simulink model "massgyro_plant"  (R2019b)
settings: Solver=VariableStepAuto  StartTime=0.0  StopTime=62  RelTol=1e-5
values from neighbouring files (symbols this model uses):
  c = 0.2    [PlantParams.mat]    (also in params.m = 0.1)
  dtheta1 = 41.8879020479    [PlantParams.mat]    (also in params.m)
  Eo = 0    [PlantParams.mat]    (also in params.m)
  g = 9.81    [PlantParams.mat]    (also in params.m)
  Id = 0.0148    [PlantParams.mat]    (also in params.m)
  J1 = 0.13138281053    [PlantParams.mat]    (also in params.m = 0.1314)
  Jz_bar = 0.0130765    [PlantParams.mat]    (also in params.m = 0.0131)
  k = 0.2    [PlantParams.mat]    (also in params.m)
  lcg = 0.269778481013    [PlantParams.mat]    (also in params.m = 0.2698)
  m = 0.158    [PlantParams.mat]    (also in params.m)
  rh = 0.37    [PlantParams.mat]    (also in params.m)
settings Model: Creator=Nilpa  LastModifiedBy=Nilpa
settings SolverCC: AlgebraicLoopSolver=LineSearch

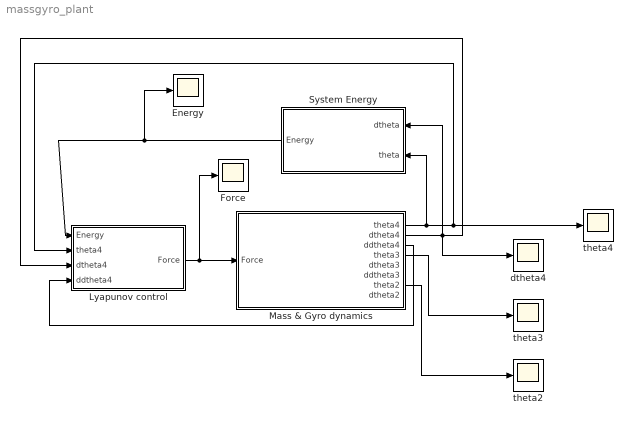
== system massgyro_plant ==
  Energy : Scope
  Force : Scope
  Lyapunov control : Subsystem
  Mass & Gyro dynamics : Subsystem
  System Energy : Subsystem
  dtheta4 : Scope
  theta2 : Scope
  theta3 : Scope
  theta4 : Scope
  wires:
  Mass & Gyro dynamics/1(theta4) -> theta4/1, Lyapunov control/2(theta4), System Energy/2(theta)
  Mass & Gyro dynamics/2(dtheta4) -> dtheta4/1, Lyapunov control/3(dtheta4), System Energy/1(dtheta)
  System Energy/1(Energy) -> Energy/1, Lyapunov control/1(Energy)
  Mass & Gyro dynamics/3(ddtheta4) -> Lyapunov control/4(ddtheta4)
  Lyapunov control/1(Force) -> Force/1, Mass & Gyro dynamics/1(Force)
  Mass & Gyro dynamics/4(theta3) -> theta3/1
  Mass & Gyro dynamics/7(theta2) -> theta2/1

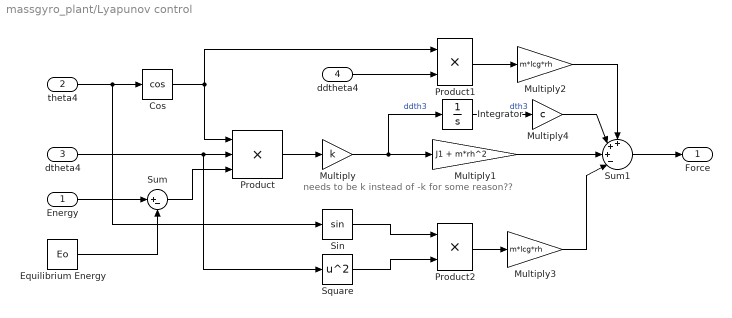
== system massgyro_plant/Lyapunov control ==
  note: needs to be k instead of -k for some reason??
  Energy : Inport
  theta4 : Inport  Port=2
  dtheta4 : Inport  Port=3
  ddtheta4 : Inport  Port=4
  Cos : Trigonometry  Operator=cos
  Equilibrium Energy : Constant  Value=Eo
  Integrator : Integrator
  Multiply : Gain  Gain=k
  Multiply1 : Gain  Gain=J1 + m*rh^2
  Multiply2 : Gain  Gain=m*lcg*rh
  Multiply3 : Gain  Gain=m*lcg*rh
  Multiply4 : Gain  Gain=c
  Product : Product  Inputs=3
  Product1 : Product
  Product2 : Product
  Sin : Trigonometry
  Square : Math  Operator=square  SignedPower=off  SaturateOnIntegerOverflow=on
  Sum : Sum  Inputs=|+-
  Sum1 : Sum  Inputs=+++-|
  Force : Outport
  wires:
  Product/1 -> Multiply/1
  theta4/1 -> Cos/1, Sin/1
  Cos/1 -> Product/1, Product1/1
  dtheta4/1 -> Product/2, Square/1
  Energy/1 -> Sum/1
  Sum/1 -> Product/3
  Equilibrium Energy/1 -> Sum/2
  Multiply/1 -> Integrator/1, Multiply1/1  "ddth3"
  Multiply1/1 -> Sum1/3
  Sum1/1 -> Force/1
  Product1/1 -> Multiply2/1
  Multiply2/1 -> Sum1/1
  Sin/1 -> Product2/1
  Square/1 -> Product2/2
  Product2/1 -> Multiply3/1
  Multiply3/1 -> Sum1/4
  ddtheta4/1 -> Product1/2
  Integrator/1 -> Multiply4/1  "dth3"
  Multiply4/1 -> Sum1/2

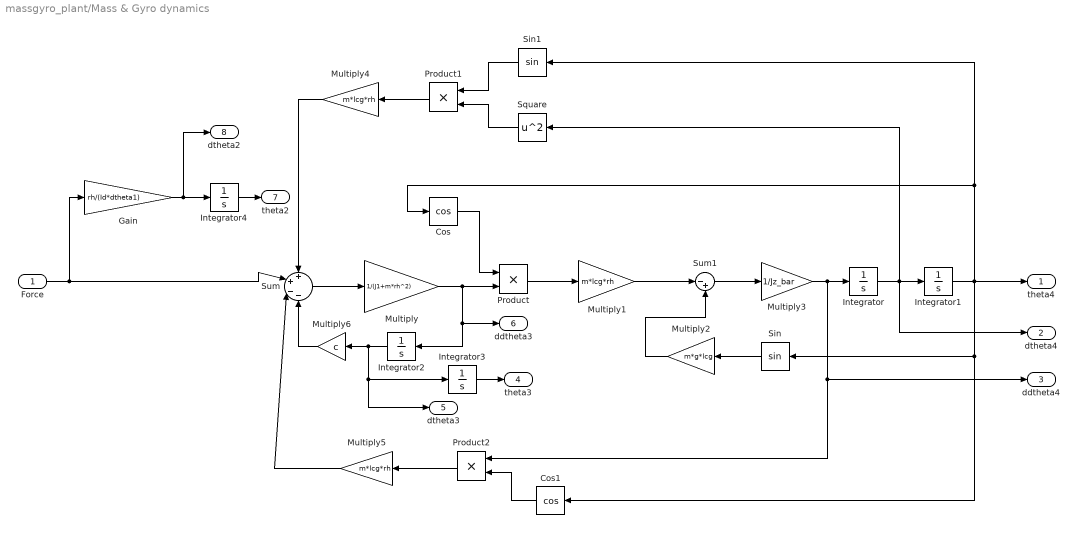
== system massgyro_plant/Mass & Gyro dynamics ==
  Force : Inport
  Cos : Trigonometry  Operator=cos
  Cos1 : Trigonometry  Operator=cos
  Gain : Gain  Gain=rh/(Id*dtheta1)
  Integrator{,2..4} (4 alike) : Integrator
  Integrator1 : Integrator  InitialCondition=pi-0.2
  Multiply : Gain  Gain=1/(J1+m*rh^2)
  Multiply1 : Gain  Gain=m*lcg*rh
  Multiply2 : Gain  Gain=m*g*lcg
  Multiply3 : Gain  Gain=1/Jz_bar
  Multiply4 : Gain  Gain=m*lcg*rh
  Multiply5 : Gain  Gain=m*lcg*rh
  Multiply6 : Gain  Gain=c
  Product : Product
  Product1 : Product
  Product2 : Product
  Sin : Trigonometry
  Sin1 : Trigonometry
  Square : Math  Operator=square  SignedPower=off  SaturateOnIntegerOverflow=on
  Sum : Sum  Inputs=++--
  Sum1 : Sum  Inputs=|-+
  theta4 : Outport
  dtheta4 : Outport  Port=2
  ddtheta4 : Outport  Port=3
  theta3 : Outport  Port=4
  dtheta3 : Outport  Port=5
  ddtheta3 : Outport  Port=6
  theta2 : Outport  Port=7
  dtheta2 : Outport  Port=8
  wires:
  Force/1 -> Sum/2, Gain/1
  Sum/1 -> Multiply/1
  Multiply/1 -> Integrator2/1, ddtheta3/1, Product/2
  Cos/1 -> Product/1
  Product/1 -> Multiply1/1
  Multiply1/1 -> Sum1/1
  Sin/1 -> Multiply2/1
  Multiply2/1 -> Sum1/2
  Sum1/1 -> Multiply3/1
  Multiply3/1 -> ddtheta4/1, Product2/1, Integrator/1
  Integrator/1 -> dtheta4/1, Square/1, Integrator1/1
  Integrator1/1 -> Cos1/1, Sin/1, theta4/1, Cos/1, Sin1/1
  Product1/1 -> Multiply4/1
  Multiply4/1 -> Sum/1
  Sin1/1 -> Product1/1
  Square/1 -> Product1/2
  Product2/1 -> Multiply5/1
  Multiply5/1 -> Sum/3
  Cos1/1 -> Product2/2
  Integrator2/1 -> Multiply6/1, dtheta3/1, Integrator3/1
  Multiply6/1 -> Sum/4
  Integrator3/1 -> theta3/1
  Gain/1 -> dtheta2/1, Integrator4/1
  Integrator4/1 -> theta2/1

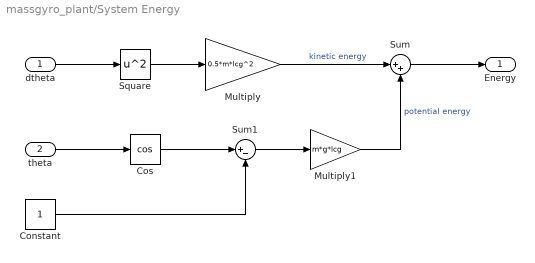
== system massgyro_plant/System Energy ==
  dtheta : Inport
  theta : Inport  Port=2
  Constant : Constant
  Cos : Trigonometry  Operator=cos
  Multiply : Gain  Gain=0.5*m*lcg^2
  Multiply1 : Gain  Gain=m*g*lcg
  Square : Math  Operator=square  SignedPower=off  SaturateOnIntegerOverflow=on
  Sum : Sum  Inputs=|++
  Sum1 : Sum  Inputs=|+-
  Energy : Outport
  wires:
  Sum/1 -> Energy/1
  Multiply/1 -> Sum/1  "kinetic energy"
  Square/1 -> Multiply/1
  dtheta/1 -> Square/1
  Constant/1 -> Sum1/2
  Cos/1 -> Sum1/1
  theta/1 -> Cos/1
  Sum1/1 -> Multiply1/1
  Multiply1/1 -> Sum/2  "potential energy"
